simulink model "Q56"  (R2023a)
settings: Solver=VariableStepAuto  StartTime=0.0  StopTime=10  MaxStep=0.001  RelTol=1e-3
settings Model: Creator=Physics Library  LastModifiedBy=Physics Library

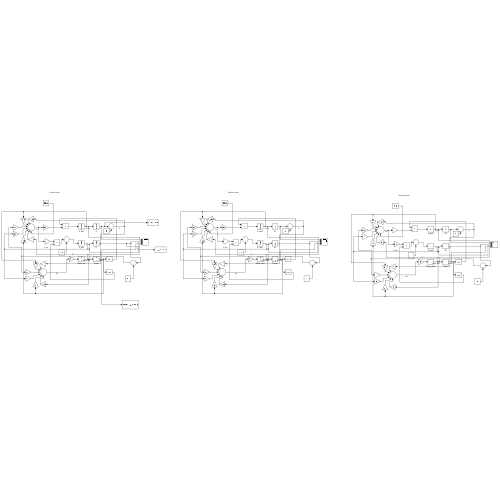
[thumbnail: Simulink's stored preview of the top-level diagram]
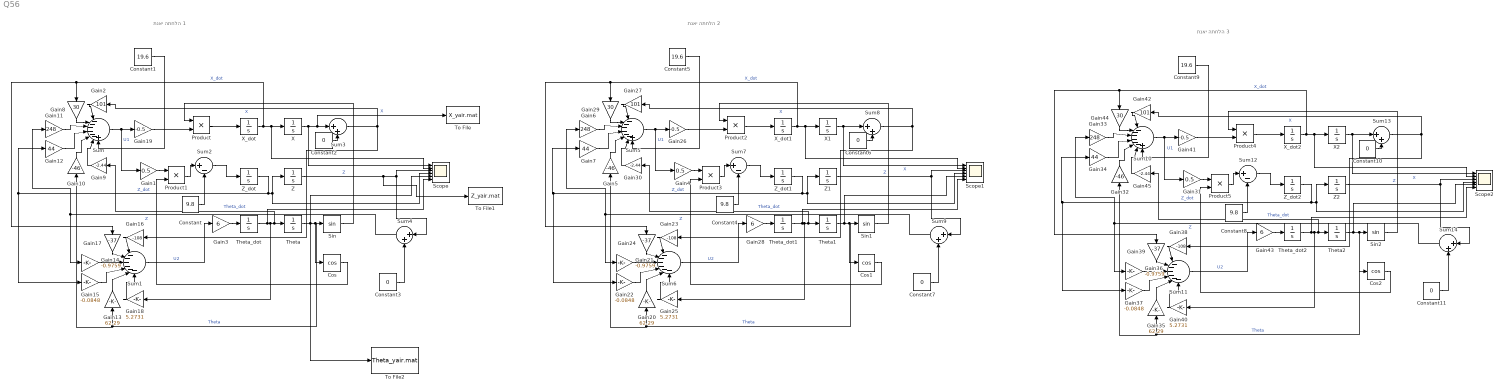
== system Q56 ==
  note: תנאי התחלה 1
  note: תנאי התחלה 2
  note: תנאי התחלה 3
  Constant : Constant  Value=9.8
  Constant1 : Constant  Value=19.6
  Constant{2..3,6..7,10..11} (6 alike) : Constant  Value=0
  Constant4 : Constant  Value=9.8
  Constant5 : Constant  Value=19.6
  Constant8 : Constant  Value=9.8
  Constant9 : Constant  Value=19.6
  Cos : Trigonometry  Operator=cos
  Cos1 : Trigonometry  Operator=cos
  Cos2 : Trigonometry  Operator=cos
  Gain1 : Gain  Gain=0.5
  Gain10 : Gain  Gain=-46
  Gain11 : Gain  Gain=248
  Gain12 : Gain  Gain=44
  Gain13 : Gain  Gain=62.29
  Gain14 : Gain  Gain=-0.9759
  Gain15 : Gain  Gain=-0.0848
  Gain16 : Gain  Gain=-108
  Gain17 : Gain  Gain=-37
  Gain18 : Gain  Gain=5.2731
  Gain19 : Gain  Gain=-0.5
  Gain2 : Gain  Gain=101
  Gain20 : Gain  Gain=62.29
  Gain21 : Gain  Gain=-0.9759
  Gain22 : Gain  Gain=-0.0848
  Gain23 : Gain  Gain=-108
  Gain24 : Gain  Gain=-37
  Gain25 : Gain  Gain=5.2731
  Gain26 : Gain  Gain=-0.5
  Gain27 : Gain  Gain=101
  Gain28 : Gain  Gain=6
  Gain29 : Gain  Gain=30
  Gain3 : Gain  Gain=6
  Gain30 : Gain  Gain=-2.44
  Gain31 : Gain  Gain=0.5
  Gain32 : Gain  Gain=-46
  Gain33 : Gain  Gain=248
  Gain34 : Gain  Gain=44
  Gain35 : Gain  Gain=62.29
  Gain36 : Gain  Gain=-0.9759
  Gain37 : Gain  Gain=-0.0848
  Gain38 : Gain  Gain=-108
  Gain39 : Gain  Gain=-37
  Gain4 : Gain  Gain=0.5
  Gain40 : Gain  Gain=5.2731
  Gain41 : Gain  Gain=-0.5
  Gain42 : Gain  Gain=101
  Gain43 : Gain  Gain=6
  Gain44 : Gain  Gain=30
  Gain45 : Gain  Gain=-2.44
  Gain5 : Gain  Gain=-46
  Gain6 : Gain  Gain=248
  Gain7 : Gain  Gain=44
  Gain8 : Gain  Gain=30
  Gain9 : Gain  Gain=-2.44
  Product{,1..5} (6 alike) : Product
  Scope : Scope  NumInputPorts=6
  Scope1 : Scope  NumInputPorts=6
  Scope2 : Scope  NumInputPorts=6
  Sin : Trigonometry
  Sin1 : Trigonometry
  Sin2 : Trigonometry
  Sum : Sum  Inputs=|------+
  Sum1 : Sum  Inputs=|------
  Sum10 : Sum  Inputs=|------+
  Sum11 : Sum  Inputs=|------
  Sum12 : Sum  Inputs=|+-
  Sum{3..4,8..9,13..14} (6 alike) : Sum  Inputs=|++
  Sum2 : Sum  Inputs=|+-
  Sum5 : Sum  Inputs=|------+
  Sum6 : Sum  Inputs=|------
  Sum7 : Sum  Inputs=|+-
  Theta : Integrator
  Theta1 : Integrator  InitialCondition=0.1
  Theta2 : Integrator
  Theta_dot : Integrator
  Theta_dot1 : Integrator
  Theta_dot2 : Integrator
  To File : ToFile  Filename=X_yair.mat  SaveFormat=Timeseries
  To File1 : ToFile  Filename=Z_yair.mat  SaveFormat=Timeseries
  To File2 : ToFile  Filename=Theta_yair.mat  SaveFormat=Timeseries
  X : Integrator
  X1 : Integrator
  X2 : Integrator  InitialCondition=0.1
  X_dot : Integrator
  X_dot1 : Integrator
  X_dot2 : Integrator
  Z : Integrator
  Z1 : Integrator
  Z2 : Integrator
  Z_dot : Integrator
  Z_dot1 : Integrator
  Z_dot2 : Integrator
  wires:
  Sum3/1 -> Gain16/1, Gain2/1  "X"
  X_dot/1 -> Gain8/1, Gain17/1, X/1, Scope/2  "X_dot"
  Sum4/1 -> Gain11/1, Gain14/1  "Z"
  Z_dot/1 -> Gain12/1, Gain15/1, Z/1, Scope/4  "Z_dot"
  Theta/1 -> To File2/1, Gain10/1, Gain13/1, Cos/1, Sin/1, Scope/5  "Theta"
  Theta_dot/1 -> Gain18/1, Gain9/1, Theta/1, Scope/6  "Theta_dot"
  Gain2/1 -> Sum/1
  Gain8/1 -> Sum/2
  Gain9/1 -> Sum/6
  Gain10/1 -> Sum/5
  Gain11/1 -> Sum/3
  Gain12/1 -> Sum/4
  Sum2/1 -> Z_dot/1
  Gain15/1 -> Sum1/4
  Gain17/1 -> Sum1/2
  Gain18/1 -> Sum1/6
  Gain13/1 -> Sum1/5
  Sum1/1 -> Gain3/1  "U2"
  Gain14/1 -> Sum1/3
  Gain16/1 -> Sum1/1
  Gain3/1 -> Theta_dot/1
  Sum/1 -> Gain19/1, Gain1/1  "U1"
  Gain19/1 -> Product/2
  Sin/1 -> Product/1
  Product/1 -> X_dot/1
  Gain1/1 -> Product1/1
  Cos/1 -> Product1/2
  Product1/1 -> Sum2/1
  Constant/1 -> Sum2/2
  Constant1/1 -> Sum/7
  X/1 -> To File/1, Sum3/1, Scope/1  "X"
  Constant2/1 -> Sum3/2
  Z/1 -> To File1/1, Sum4/1, Scope/3  "Z"
  Constant3/1 -> Sum4/2
  Constant6/1 -> Sum8/2
  Sum9/1 -> Gain6/1, Gain21/1  "Z"
  Sin1/1 -> Product2/1
  Cos1/1 -> Product3/2
  Z_dot1/1 -> Gain7/1, Gain22/1, Z1/1, Scope1/4  "Z_dot"
  Gain4/1 -> Product3/1
  Constant7/1 -> Sum9/2
  Z1/1 -> Sum9/1, Scope1/3  "Z"
  Gain29/1 -> Sum5/2
  Gain23/1 -> Sum6/1
  Gain26/1 -> Product2/2
  X1/1 -> Sum8/1, Scope1/1  "X"
  Gain21/1 -> Sum6/3
  Sum6/1 -> Gain28/1  "U2"
  Gain20/1 -> Sum6/5
  Sum7/1 -> Z_dot1/1
  Gain6/1 -> Sum5/3
  Gain24/1 -> Sum6/2
  Theta_dot1/1 -> Gain25/1, Gain30/1, Theta1/1, Scope1/6  "Theta_dot"
  Gain7/1 -> Sum5/4
  Gain22/1 -> Sum6/4
  Sum5/1 -> Gain26/1, Gain4/1  "U1"
  Gain30/1 -> Sum5/6
  Gain5/1 -> Sum5/5
  Gain27/1 -> Sum5/1
  Product2/1 -> X_dot1/1
  Sum8/1 -> Gain23/1, Gain27/1  "X"
  X_dot1/1 -> Gain29/1, Gain24/1, X1/1, Scope1/2  "X_dot"
  Product3/1 -> Sum7/1
  Theta1/1 -> Gain5/1, Gain20/1, Cos1/1, Sin1/1, Scope1/5  "Theta"
  Gain28/1 -> Theta_dot1/1
  Constant5/1 -> Sum5/7
  Gain25/1 -> Sum6/6
  Constant4/1 -> Sum7/2
  Constant10/1 -> Sum13/2
  Sum14/1 -> Gain33/1, Gain36/1  "Z"
  Sin2/1 -> Product4/1
  Cos2/1 -> Product5/2
  Z_dot2/1 -> Gain34/1, Gain37/1, Z2/1, Scope2/4  "Z_dot"
  Gain31/1 -> Product5/1
  Constant11/1 -> Sum14/2
  Z2/1 -> Sum14/1, Scope2/3  "Z"
  Gain44/1 -> Sum10/2
  Gain38/1 -> Sum11/1
  Gain41/1 -> Product4/2
  X2/1 -> Sum13/1, Scope2/1  "X"
  Gain36/1 -> Sum11/3
  Sum11/1 -> Gain43/1  "U2"
  Gain35/1 -> Sum11/5
  Sum12/1 -> Z_dot2/1
  Gain33/1 -> Sum10/3
  Gain39/1 -> Sum11/2
  Theta_dot2/1 -> Gain40/1, Gain45/1, Theta2/1, Scope2/6  "Theta_dot"
  Gain34/1 -> Sum10/4
  Gain37/1 -> Sum11/4
  Sum10/1 -> Gain41/1, Gain31/1  "U1"
  Gain45/1 -> Sum10/6
  Gain32/1 -> Sum10/5
  Gain42/1 -> Sum10/1
  Product4/1 -> X_dot2/1
  Sum13/1 -> Gain38/1, Gain42/1  "X"
  X_dot2/1 -> Gain44/1, Gain39/1, X2/1, Scope2/2  "X_dot"
  Product5/1 -> Sum12/1
  Theta2/1 -> Gain32/1, Gain35/1, Cos2/1, Sin2/1, Scope2/5  "Theta"
  Gain43/1 -> Theta_dot2/1
  Constant9/1 -> Sum10/7
  Gain40/1 -> Sum11/6
  Constant8/1 -> Sum12/2
